simulink subsystem "Beobachter"  (R2020a)
settings: Solver=VariableStepAuto  StartTime=0.0  StopTime=10.0  RelTol=1e-3
model mask{A=[], B=[], C=[], L=[], vT=[], xb0=[]}
  mask prompts: vT "Zeitvektor"; xb0 "Startwert"
values from neighbouring files (symbols this model uses):
  L = place(sys.A', sys.C', pole).'    [PlaceBeobachter.m]
settings Model: Creator=Tobias  LastModifiedBy=Frederik

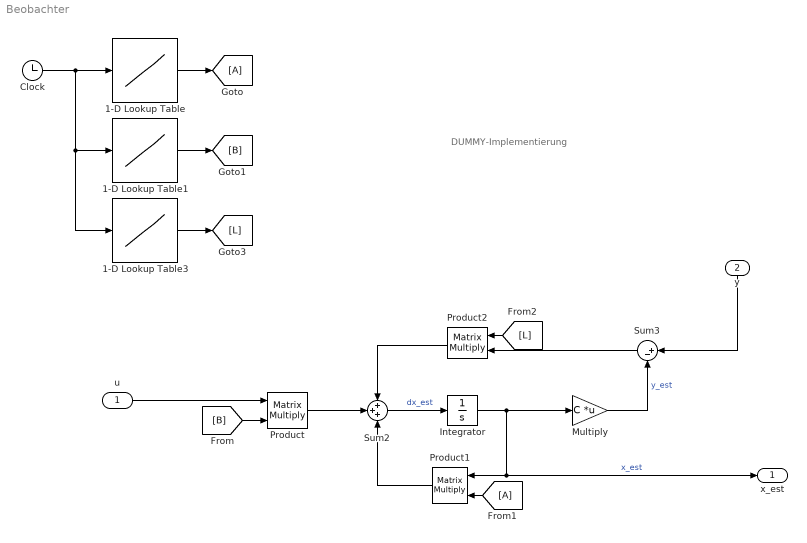
== system Beobachter ==
  note: DUMMY-Implementierung
  u : Inport
  y : Inport  Port=2
  1-D Lookup Table : Lookup_n-D  NumberOfTableDimensions=1  BreakpointsForDimension1=vT  Table=A  InternalRulePriority=Speed  RndMeth=Simplest  InputSameDT=on
  1-D Lookup Table1 : Lookup_n-D  NumberOfTableDimensions=1  BreakpointsForDimension1=vT  Table=B  InternalRulePriority=Speed  RndMeth=Simplest  InputSameDT=on
  1-D Lookup Table3 : Lookup_n-D  NumberOfTableDimensions=1  BreakpointsForDimension1=vT  Table=L  InternalRulePriority=Speed  RndMeth=Simplest  InputSameDT=on
  Clock : Clock
  Integrator : Integrator  InitialCondition=xb0
  Multiply : Gain  Gain=C  Multiplication=Matrix(K*u)
  Product : Product  Multiplication=Matrix(*)
  Product1 : Product  Multiplication=Matrix(*)
  Product2 : Product  Multiplication=Matrix(*)
  Sum2 : Sum  Inputs=+++
  Sum3 : Sum  Inputs=|+-
  x_est : Outport
  wires:
  Product/1 -> Sum2/2
  Product2/1 -> Sum2/1
  Sum2/1 -> Integrator/1  "dx_est"
  Sum3/1 -> Product2/2
  Multiply/1 -> Sum3/2  "y_est"
  y/1 -> Sum3/1
  Product1/1 -> Sum2/3
  Integrator/1 -> x_est/1, Product1/1, Multiply/1  "x_est"
  u/1 -> Product/1
  Clock/1 -> 1-D Lookup Table/1, 1-D Lookup Table1/1, 1-D Lookup Table3/1
  1-D Lookup Table/1 -> [A]
  1-D Lookup Table1/1 -> [B]
  1-D Lookup Table3/1 -> [L]
  [B] -> Product/2
  [A] -> Product1/2
  [L] -> Product2/1
